simulink model "Speed_2016b"  (R2019a)
settings: Solver=ode4  StartTime=0.0  StopTime=3000  FixedStep=0.1  RelTol=1e-3
model workspace (MAT data in the model file):
  k0 = Simulink.Parameter
  k0.DataType = 'auto'
  k0.Dimensions = [0 0]
undefined symbols (not defined in the file or in its folder): sigbuilder_block
libraries: fuzblock x1
settings Model: Creator=ASUS  LastModifiedBy=ASUS
settings DebuggingCC: ArithmeticOperatorsInVariantConditions=warning
settings CodeAppCC: StateflowObjectComments=on

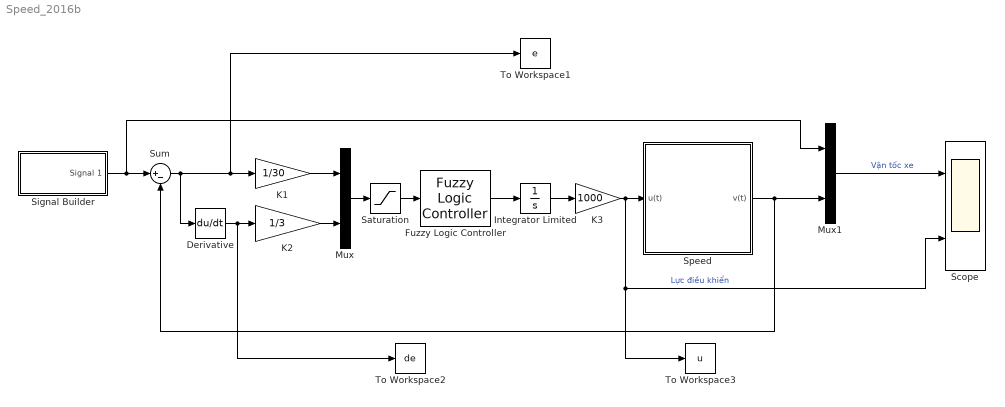
== system Speed_2016b ==
  Derivative : Derivative
  Fuzzy Logic Controller : fuzblock/Fuzzy Logic  Controller  FIS='bt2.fis'  OutputSampleNumber=101  DataType=double  FuzzifiedInputs=off  RuleFiringStrengths=off  RuleOutputs=off  AggregatedOutputs=off  SimulateUsing=Interpreted execution  OutOfRangeInputValueMessage=warning  NoRuleFiredMessage=warning  EmptyOutputFuzzySetMessage=warning
  Integrator Limited : Integrator  LimitOutput=on  UpperSaturationLimit=1  LowerSaturationLimit=-1
  K1 : Gain  Gain=1/30
  K2 : Gain  Gain=1/3
  K3 : Gain  Gain=1000
  Mux : Mux  Inputs=2
  Mux1 : Mux  Inputs=2
  Saturation : Saturate  UpperLimit=1  LowerLimit=-1
  Scope : Scope  NumInputPorts=2
  Signal Builder : Subsystem  Tag=STV Subsys  LoadFcn=sigbuilder_block('load');  StartFcn=sigbuilder_block('start');  StopFcn=sigbuilder_block('stop');  ClipboardFcn=sigbuilder_block('clipboard');  mask(Sigbuilder block){tuvar=[0:10]}
      mask help: Simulink:masks:SigbuilderBlock_MD
      mask init:
      | if ~strcmp(get_param(bdroot(gcbh),'SimulationStatus'),'stopped') tuvar = sigbuilder_block('maskInit'); end
      settings: CopyFcn=sigbuilder_block('copy');  DeleteFcn=sigbuilder_block('delete');  ModelCloseFcn=sigbuilder_block('modelClose');  PreSaveFcn=sigbuilder_block('preSave');  PauseFcn=sigbuilder_block('pause');  ContinueFcn=sigbuilder_block('continue');  NameChangeFcn=sigbuilder_block('namechange');  OpenFcn=sigbuilder_block('open',[538.8 144.6 550.8 400.2 ]);  CloseFcn=sigbuilder_block('close');
      mask Display: plot(0, 0, 100, 100,[2, 2, 32, 32, 2], [68, 8, 8, 68, 68],[32, 2], [38, 38], [32, 19, 2],[53, 60, 44], [32, 17, 17, 2],[16, 16, 31, 31]);txt = getActiveGroup(gcbh);text(2, 100, txt,'verticalAlignment', 'top');
  Speed : Subsystem  mask{Ap=0.3, d=100, t=0.2, m=1300}
      mask Display: image(imread('bt2.png'))
  Sum : Sum  Inputs=|+-
  To Workspace1 : ToWorkspace  VariableName=e  SampleTime=-1
  To Workspace2 : ToWorkspace  VariableName=de  SampleTime=-1
  To Workspace3 : ToWorkspace  VariableName=u  SampleTime=-1
  wires:
  K3/1 -> To Workspace3/1, Scope/2, Speed/1(u(t))  "Lực điều khiển"
  Saturation/1 -> Fuzzy Logic Controller/1
  Mux/1 -> Saturation/1
  Derivative/1 -> To Workspace2/1, K2/1
  Sum/1 -> To Workspace1/1, K1/1, Derivative/1
  Signal Builder/1(Signal 1) -> Mux1/1, Sum/1
  Mux1/1 -> Scope/1  "Vận tốc xe"
  Integrator Limited/1 -> K3/1
  Fuzzy Logic Controller/1 -> Integrator Limited/1
  Speed/1(v(t)) -> Mux1/2, Sum/2
  K1/1 -> Mux/1
  K2/1 -> Mux/2

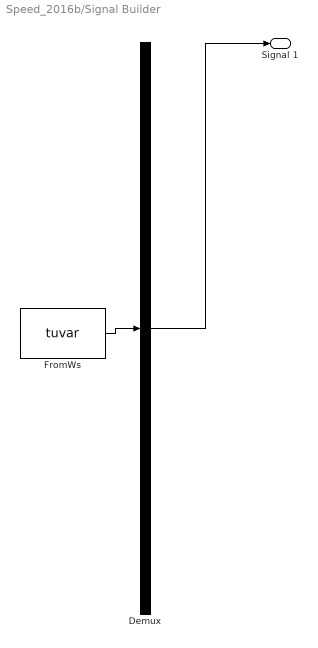
== system Speed_2016b/Signal Builder ==
  Demux : Demux  Tag=STV Demux  Outputs=1
  FromWs : FromWorkspace  Tag=STV FromWs  VariableName=tuvar  SampleTime=0
      SigBuilderData=|
      | common.afterFinalStr = 'Extrapolate'
      | common.sampleTime = 0
      | dataSet.timeRange = [0 3000]
      | dataSet.name = 'Group 1'
      | sbobj.Groups.Name = 'Group 1'
      | sbobj.Groups.Signals.Name = 'Signal 1'
      | sbobj.Groups.Signals.XData = [0 130 130 280 280 510 510 650 650 900 900 1120 1120 1435 1435 1800 1800 2115 2115 2380 2380 2700 2700 3000]
      | sbobj.Groups.Signals.YData = [28 28 24 24 20 20 17 17 0 0 5 5 2 2 8 8 14 14 20 20 11 11 24 24]
      | sbobj.Groups.TimeRange = [0 3000]
  Signal 1 : Outport  Tag=STV Outport
  wires:
  Demux/1 -> Signal 1/1
  FromWs/1 -> Demux/1

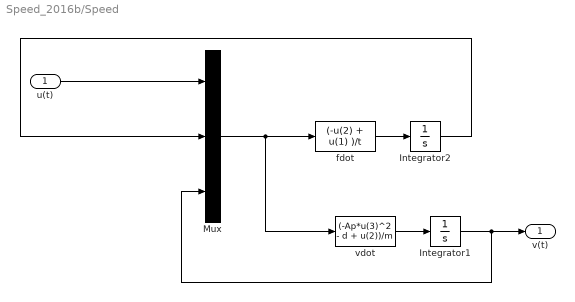
== system Speed_2016b/Speed ==
  u(t) : Inport
  Integrator1 : Integrator
  Integrator2 : Integrator
  Mux : Mux  Inputs=3
  fdot : Fcn  Expr=(-u(2) + u(1) )/t
  vdot : Fcn  Expr=(-Ap*u(3)^2 - d + u(2))/m
  v(t) : Outport
  wires:
  fdot/1 -> Integrator2/1
  Integrator2/1 -> Mux/2
  Mux/1 -> vdot/1, fdot/1
  u(t)/1 -> Mux/1
  Integrator1/1 -> Mux/3, v(t)/1
  vdot/1 -> Integrator1/1
